simulink model "modelagem"  (R2022b)
settings: Solver=VariableStepAuto  StartTime=0.0  StopTime=10  RelTol=1e-3
StopFcn:
  | q = out.logsout{2}.Values;
  | wc = out.logsout{1}.Values;
  | figure(1)
  | plot(q.Time,q.Data)
  | 
  | hold off
  | figure(2)
  | plot(wc.Time,wc.Data)
  | legend("\omega_x","\omega_y","\omega_z")
  | ylabel("Velocidade Angular [rad/s]")
  | xlabel("Tempo [s]")
values from neighbouring files (symbols this model uses):
  b = 17.03*10^(-6)    (= 1.703e-05)    [modelagem_script.m]
  g = [0;0;-9.81]    [modelagem_script.m]
  Ic = [0.01008 -0.00309375 -0.00309375 ... (first row only)    [modelagem_script.m]
  mc = 0.55    [modelagem_script.m]
  q00 = [cos(phi_u/2);e_u*sin(phi_u/2)]    [modelagem_script.m]
  rc = [0.0954545;0.0954545;0.0954545]    [modelagem_script.m]
  Tau = [0;0;0]    [modelagem_script.m]
  w00 = [0;0;0]    [modelagem_script.m]
libraries: vrlib x2
settings Model: Creator=guimi  LastModifiedBy=guimi

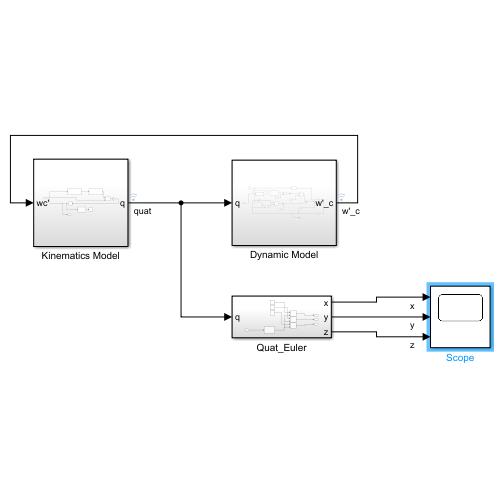
[thumbnail: Simulink's stored preview of the top-level diagram]
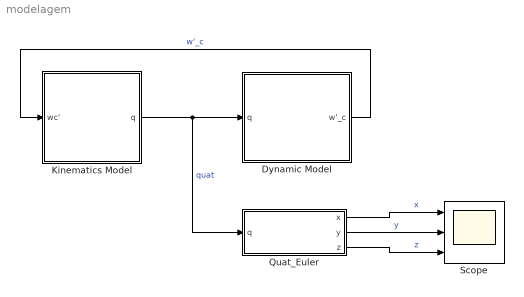
== system modelagem ==
  Dynamic Model : Subsystem
  Kinematics Model : Subsystem
  Quat_Euler : Subsystem
  Scope : Scope  NumInputPorts=3
  wires:
  Kinematics Model/1(q) -> Quat_Euler/1(q), Dynamic Model/1(q)  "quat"
  Dynamic Model/1(w'_c) -> Kinematics Model/1(wc')  "w'_c"
  Quat_Euler/1(x) -> Scope/1  "x"
  Quat_Euler/2(y) -> Scope/2  "y"
  Quat_Euler/3(z) -> Scope/3  "z"

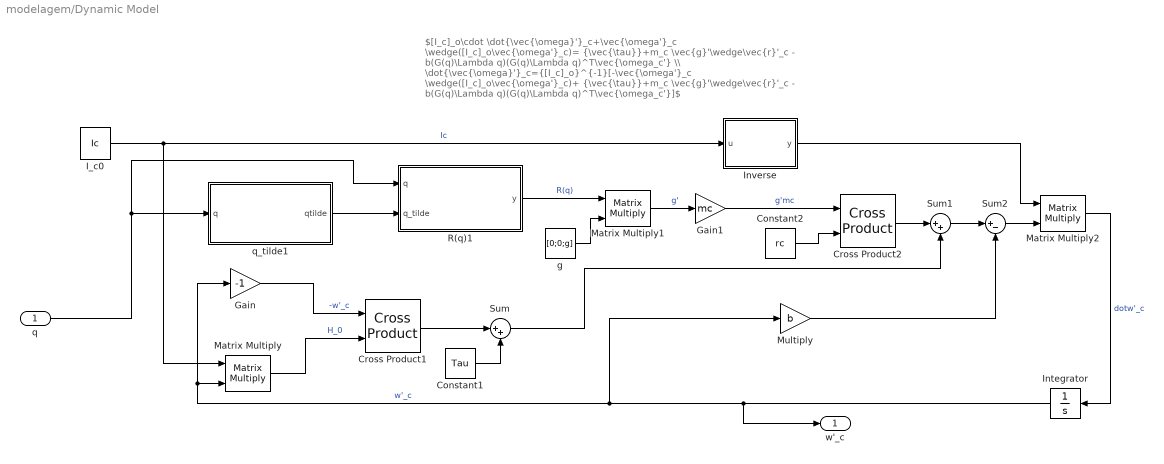
== system modelagem/Dynamic Model ==
  note: $[I_c]_o\cdot \dot{\vec{\omega}'}_c+\vec{\omega'}_c \wedge([I_c]_o\vec{\omega'}_c)= {\vec{\tau}}+m_c \vec{g}'\wedge\vec{r}'_c - b(G(q)\Lambda q)(G(q)\Lambda q)^T\vec{\omega_c'} \\ \dot{\vec{\omega}'}_c={[I_c]_o}^{-1}[-\vec{\omega'}_c \wedge([I_c]_o\vec{\omega'}_c)+ {\vec{\tau}}+m_c \vec{g}'\wedge\vec{r}'_c - b(G(q)\Lambda q)(G(q)\Lambda q)^T\vec{\omega_c'}]$
  q : Inport
  Constant1 : Constant  Value=Tau
  Constant2 : Constant  Value=rc
  Cross Product1 : vrlib/Utilities/Cross Product
  Cross Product2 : vrlib/Utilities/Cross Product
  Gain : Gain  Gain=-1
  Gain1 : Gain  Gain=mc
  I_c0 : Constant  Value=Ic
  Integrator : Integrator  InitialCondition=w00
  Inverse : MATLAB Function  TreatAsAtomicUnit=on
  Matrix Multiply : Product  Multiplication=Matrix(*)
  Matrix Multiply1 : Product  Multiplication=Matrix(*)
  Matrix Multiply2 : Product  Multiplication=Matrix(*)
  Multiply : Gain  Gain=b
  R(q)1 : MATLAB Function  TreatAsAtomicUnit=on
  Sum : Sum  Inputs=|++
  Sum1 : Sum  Inputs=|++
  Sum2 : Sum  Inputs=|+-
  g : Constant  Value=[0;0;g]
  q_tilde1 : Subsystem
  w'_c : Outport
  wires:
  q_tilde1/1(qtilde) -> R(q)1/2(q_tilde)
  I_c0/1 -> Inverse/1(u), Matrix Multiply/1  "Ic"
  Integrator/1 -> Matrix Multiply/2, Gain/1, Multiply/1, w'_c/1  "w'_c"
  Matrix Multiply/1 -> Cross Product1/2  "H_0"
  Gain/1 -> Cross Product1/1  "-w'_c"
  Cross Product1/1 -> Sum/1
  Constant1/1 -> Sum/2
  q/1 -> R(q)1/1(q), q_tilde1/1(q)
  R(q)1/1(y) -> Matrix Multiply1/1  "R(q)"
  g/1 -> Matrix Multiply1/2
  Matrix Multiply1/1 -> Gain1/1  "g'"
  Gain1/1 -> Cross Product2/1  "g'mc"
  Constant2/1 -> Cross Product2/2
  Cross Product2/1 -> Sum1/1
  Sum/1 -> Sum1/2
  Sum1/1 -> Sum2/1
  Multiply/1 -> Sum2/2
  Sum2/1 -> Matrix Multiply2/2
  Inverse/1(y) -> Matrix Multiply2/1
  Matrix Multiply2/1 -> Integrator/1  "dotw'_c"

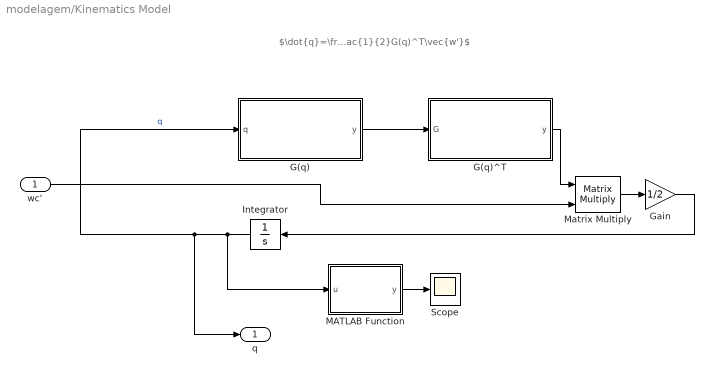
== system modelagem/Kinematics Model ==
  note: $\dot{q}=\frac{1}{2}G(q)^T\vec{w'}$
  wc' : Inport
  G(q) : MATLAB Function  TreatAsAtomicUnit=on
  G(q)^T : MATLAB Function  TreatAsAtomicUnit=on
  Gain : Gain  Gain=1/2
  Integrator : Integrator  InitialCondition=q00
  MATLAB Function : MATLAB Function  TreatAsAtomicUnit=on
  Matrix Multiply : Product  Multiplication=Matrix(*)
  Scope : Scope
  q : Outport
  wires:
  G(q)/1(y) -> G(q)^T/1(G)
  Gain/1 -> Integrator/1
  wc'/1 -> Matrix Multiply/2
  G(q)^T/1(y) -> Matrix Multiply/1
  Integrator/1 -> MATLAB Function/1(u), q/1, G(q)/1(q)  "q"
  Matrix Multiply/1 -> Gain/1
  MATLAB Function/1(y) -> Scope/1

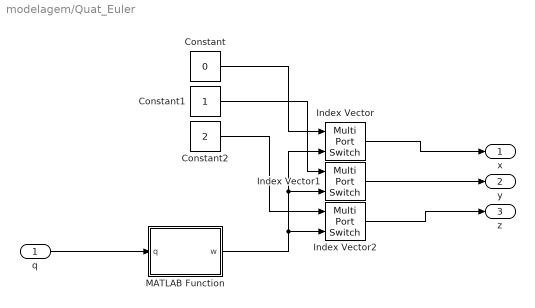
== system modelagem/Quat_Euler ==
  q : Inport
  Constant : Constant  Value=0
  Constant1 : Constant
  Constant2 : Constant  Value=2
  Index Vector : MultiPortSwitch  DataPortOrder=Zero-based contiguous  Inputs=1  zeroidx=on  SaturateOnIntegerOverflow=off  InputSameDT=off
  Index Vector1 : MultiPortSwitch  DataPortOrder=Zero-based contiguous  Inputs=1  zeroidx=on  SaturateOnIntegerOverflow=off  InputSameDT=off
  Index Vector2 : MultiPortSwitch  DataPortOrder=Zero-based contiguous  Inputs=1  zeroidx=on  SaturateOnIntegerOverflow=off  InputSameDT=off
  MATLAB Function : MATLAB Function  TreatAsAtomicUnit=on
  x : Outport
  y : Outport  Port=2
  z : Outport  Port=3
  wires:
  q/1 -> MATLAB Function/1(q)
  MATLAB Function/1(w) -> Index Vector/2, Index Vector1/2, Index Vector2/2
  Constant2/1 -> Index Vector2/1
  Constant1/1 -> Index Vector1/1
  Constant/1 -> Index Vector/1
  Index Vector/1 -> x/1
  Index Vector1/1 -> y/1
  Index Vector2/1 -> z/1

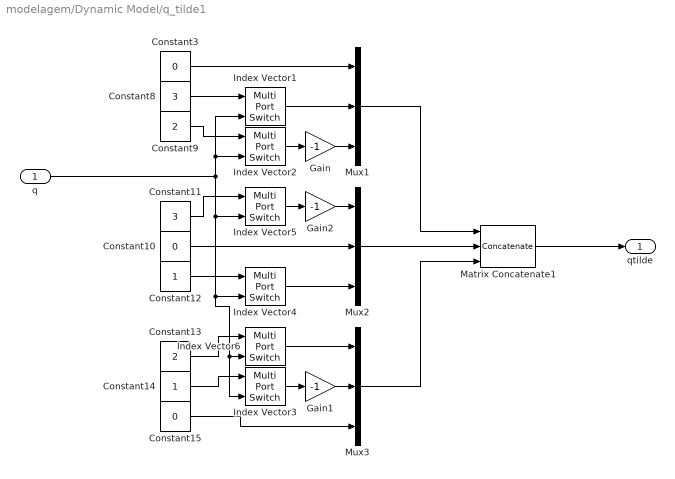
== system modelagem/Dynamic Model/q_tilde1 ==
  q : Inport
  Constant10 : Constant  Value=0
  Constant11 : Constant  Value=3
  Constant12 : Constant
  Constant13 : Constant  Value=2
  Constant14 : Constant
  Constant15 : Constant  Value=0
  Constant3 : Constant  Value=0
  Constant8 : Constant  Value=3
  Constant9 : Constant  Value=2
  Gain : Gain  Gain=-1
  Gain1 : Gain  Gain=-1
  Gain2 : Gain  Gain=-1
  Index Vector{1..6} (6 alike) : MultiPortSwitch  DataPortOrder=Zero-based contiguous  Inputs=1  zeroidx=on  SaturateOnIntegerOverflow=off  InputSameDT=off
  Matrix Concatenate1 : Concatenate  NumInputs=3  Mode=Multidimensional array  ConcatenateDimension=2
  Mux1 : Mux  Inputs=3
  Mux2 : Mux  Inputs=3
  Mux3 : Mux  Inputs=3
  qtilde : Outport
  wires:
  q/1 -> Index Vector5/2, Index Vector3/2, Index Vector6/2, Index Vector4/2, Index Vector1/2, Index Vector2/2
  Constant3/1 -> Mux1/1
  Constant8/1 -> Index Vector1/1
  Index Vector1/1 -> Mux1/2
  Constant9/1 -> Index Vector2/1
  Index Vector2/1 -> Gain/1
  Gain/1 -> Mux1/3
  Index Vector4/1 -> Mux2/3
  Constant10/1 -> Mux2/2
  Index Vector5/1 -> Gain2/1
  Gain2/1 -> Mux2/1
  Constant11/1 -> Index Vector5/1
  Constant12/1 -> Index Vector4/1
  Index Vector6/1 -> Mux3/1
  Constant15/1 -> Mux3/3
  Constant13/1 -> Index Vector6/1
  Constant14/1 -> Index Vector3/1
  Index Vector3/1 -> Gain1/1
  Gain1/1 -> Mux3/2
  Mux2/1 -> Matrix Concatenate1/2
  Mux1/1 -> Matrix Concatenate1/1
  Mux3/1 -> Matrix Concatenate1/3
  Matrix Concatenate1/1 -> qtilde/1

== matlab function modelagem/Dynamic Model/Inverse ==
  data: u input; y output
function y = fcn(u)
    
y = inv(u);

== matlab function modelagem/Quat_Euler/MATLAB Function ==
  data: q input; w output
function w = fcn(q)

    t0 = 2 * (q(1)*q(2)+q(3)*q(4));
    t1 = 1 - 2 * (q(2)*q(2)+q(3)*q(3));
    x = atan2(t0,t1);

    t2 = 2*(q(1)*q(3)-q(2)*q(4));
    if t2 > 1
        t22 = 1;
    elseif t2 < -1
        t22 = -1;
    else
        t22 = t2;
    end
    y = asin(t22);

    t3 = 2 * (q(1)*q(4)+q(2)*q(3));
    t4 = 1 - 2 * (q(3)*q(3)+q(4)*q(4));
    z = atan2(t3,t4);

w = [x;y;z];

== matlab function modelagem/Kinematics Model/G(q) ==
  data: q input; y output
function y = fcn(q)
    y = [-q(2) q(1) q(4) -q(3); -q(3) -q(4) q(1) q(2); -q(4) q(3) -q(2) q(1)];  
end

== matlab function modelagem/Kinematics Model/G(q)^T ==
  data: G input; y output
function y = fcn(G)
    y = G.';  
end

== matlab function modelagem/Kinematics Model/MATLAB Function ==
  data: u input; y output
function y = norma(u)

y = norm(u);

== matlab function modelagem/Dynamic Model/R(q)1 ==
  data: q input; y output; q_tilde input
function y = fcn(q,q_tilde)
    I = eye(3);
    qi = [q(2),q(3),q(4)];
    qT = qi.';
    y = (q(1)*I+qi*qT+2*q(1)*q_tilde+q_tilde*q_tilde);
end
